simulink model "InjVlv_CalcET1"  (R2016b)
settings: configuration reference "CodeGenConfigSet" (kept outside this file)
values from neighbouring files (symbols this model uses):
  InjVlv_pMin_C = Calibration.Parameter    [init_InjVlv_CalcET.m]    (also in init_InjVlv_CalcET_SIL.m = Simulink.Parameter)
  InjVlv_pMin_CUR = Calibration.Parameter    [init_InjVlv_CalcET.m]    (also in init_InjVlv_CalcET_SIL.m = Simulink.Parameter)
  InjVlv_pMin_CURX = Calibration.Parameter    [init_InjVlv_CalcET.m]    (also in init_InjVlv_CalcET_SIL.m = Simulink.Parameter)
  InjVlv_qMI1Min_CUR = Calibration.Parameter    [init_InjVlv_CalcET.m]    (also in init_InjVlv_CalcET_SIL.m = Simulink.Parameter)
  InjVlv_qMI1Min_CURX = Calibration.Parameter    [init_InjVlv_CalcET.m]    (also in init_InjVlv_CalcET_SIL.m = Simulink.Parameter)
  InjVlv_qPiI1Min_CUR = Calibration.Parameter    [init_InjVlv_CalcET.m]    (also in init_InjVlv_CalcET_SIL.m = Simulink.Parameter)
  InjVlv_qPiI1Min_CURX = Calibration.Parameter    [init_InjVlv_CalcET.m]    (also in init_InjVlv_CalcET_SIL.m = Simulink.Parameter)
  InjVlv_qPiI2Min_CUR = Calibration.Parameter    [init_InjVlv_CalcET.m]    (also in init_InjVlv_CalcET_SIL.m = Simulink.Parameter)
  InjVlv_qPiI2Min_CURX = Calibration.Parameter    [init_InjVlv_CalcET.m]    (also in init_InjVlv_CalcET_SIL.m = Simulink.Parameter)
  InjVlv_qPoI2Min_CUR = Calibration.Parameter    [init_InjVlv_CalcET.m]    (also in init_InjVlv_CalcET_SIL.m = Simulink.Parameter)
  InjVlv_qPoI2Min_CURX = Calibration.Parameter    [init_InjVlv_CalcET.m]    (also in init_InjVlv_CalcET_SIL.m = Simulink.Parameter)
  InjVlv_tiCloseDelay_MAP = Calibration.Parameter    [init_InjVlv_CalcET.m]    (also in init_InjVlv_CalcET_SIL.m = Simulink.Parameter)
  InjVlv_tiCloseDelay_MAPX = Calibration.Parameter    [init_InjVlv_CalcET.m]    (also in init_InjVlv_CalcET_SIL.m = Simulink.Parameter)
  InjVlv_tiCloseDelay_MAPY = Calibration.Parameter    [init_InjVlv_CalcET.m]    (also in init_InjVlv_CalcET_SIL.m = Simulink.Parameter)
  InjVlv_tiDiffMin_MAP = Calibration.Parameter    [init_InjVlv_CalcET.m]    (also in init_InjVlv_CalcET_SIL.m = Simulink.Parameter)
  InjVlv_tiDiffMin_MAPX = Calibration.Parameter    [init_InjVlv_CalcET.m]    (also in init_InjVlv_CalcET_SIL.m = Simulink.Parameter)
  InjVlv_tiDiffMin_MAPY = Calibration.Parameter    [init_InjVlv_CalcET.m]    (also in init_InjVlv_CalcET_SIL.m = Simulink.Parameter)
  InjVlv_tiET_MAP = Calibration.Parameter    [init_InjVlv_CalcET.m]    (also in init_InjVlv_CalcET_SIL.m = Simulink.Parameter)
  InjVlv_tiET_MAPX = Calibration.Parameter    [init_InjVlv_CalcET.m]    (also in init_InjVlv_CalcET_SIL.m = Simulink.Parameter)
  InjVlv_tiET_MAPY = Calibration.Parameter    [init_InjVlv_CalcET.m]    (also in init_InjVlv_CalcET_SIL.m = Simulink.Parameter)
  InjVlv_tiOpenDelay_MAP = Calibration.Parameter    [init_InjVlv_CalcET.m]    (also in init_InjVlv_CalcET_SIL.m = Simulink.Parameter)
  InjVlv_tiOpenDelay_MAPX = Calibration.Parameter    [init_InjVlv_CalcET.m]    (also in init_InjVlv_CalcET_SIL.m = Simulink.Parameter)
  InjVlv_tiOpenDelay_MAPY = Calibration.Parameter    [init_InjVlv_CalcET.m]    (also in init_InjVlv_CalcET_SIL.m = Simulink.Parameter)
  InjVlv_tiPseElec = Calibration.Parameter    [init_InjVlv_CalcET.m]    (also in init_InjVlv_CalcET_SIL.m = Simulink.Parameter)
  SigTst_swtMI1ET_C = Calibration.Parameter    [init_InjVlv_CalcET.m]    (also in init_InjVlv_CalcET_SIL.m = Simulink.Parameter)
  SigTst_swtPiI1ET_C = Calibration.Parameter    [init_InjVlv_CalcET.m]    (also in init_InjVlv_CalcET_SIL.m = Simulink.Parameter)
  SigTst_swtPiI2ET_C = Calibration.Parameter    [init_InjVlv_CalcET.m]    (also in init_InjVlv_CalcET_SIL.m = Simulink.Parameter)
  SigTst_swtPOI2ET_C = Calibration.Parameter    [init_InjVlv_CalcET.m]    (also in init_InjVlv_CalcET_SIL.m = Simulink.Parameter)
  SigTst_tiMI1ET_C = Calibration.Parameter    [init_InjVlv_CalcET.m]    (also in init_InjVlv_CalcET_SIL.m = Simulink.Parameter)
  SigTst_tiPiI1ET_C = Calibration.Parameter    [init_InjVlv_CalcET.m]    (also in init_InjVlv_CalcET_SIL.m = Simulink.Parameter)
  SigTst_tiPiI2ET_C = Calibration.Parameter    [init_InjVlv_CalcET.m]    (also in init_InjVlv_CalcET_SIL.m = Simulink.Parameter)
  SigTst_tiPOI2ET_C = Calibration.Parameter    [init_InjVlv_CalcET.m]    (also in init_InjVlv_CalcET_SIL.m = Simulink.Parameter)
undefined symbols (not defined in the file or in its folder): CEngDst_switch_conv, Switch_conv
libraries: simulink x1
settings Model: Creator=Administrator  LastModifiedBy=mayongchao
settings ConfigSetRef: SourceLocation=Base Workspace

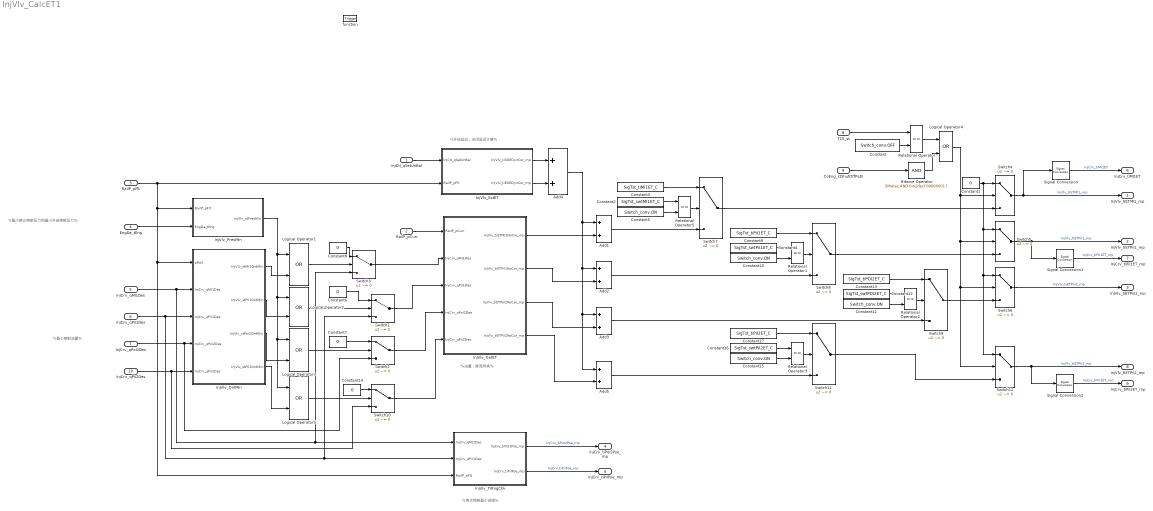
== system InjVlv_CalcET1 ==
  note: %两次喷射最小间隔%
  note: %最小喷射油量%
  note: %最小禁止喷射压力和最小开启喷射压力%
  note: %油量，脉宽转换%
  note: %开启延迟，关闭延迟计算%
  InjCtl_qSetUnBal : Inport  Tag=mg/hub  Description=Current injection quantity  OutMin=-319  OutMax=319  OutDataTypeStr=FuelMass_mg_hub
  RailP_pCurr : Inport  Tag=bar  Description=Current fuel pressure  Port=2  OutMin=0  OutMax=2500  OutDataTypeStr=RailPressure_bar
  RailP_pFlt : Inport  Tag=bar  Description=Maximum rail pressure of the last 10 sampling cycle  Port=3  OutMin=0  OutMax=2500  OutDataTypeStr=RailPressure_bar
  EngDa_tEng : Inport  Tag=deg  Description=Engine temperature  Port=4  OutMin=-1000  OutMax=1000  OutDataTypeStr=Temp_deg
  InjCrv_qMI1Des : Inport  Tag=mg/hub  Description=desired MI1 injection quantity  Port=5  OutMin=-319  OutMax=319  OutDataTypeStr=FuelMass_mg_hub
  InjCrv_qPiI1Des : Inport  Tag=mg/hub  Description=Desired PiI injection quantity  Port=6  OutMin=-319  OutMax=319  OutDataTypeStr=FuelMass_mg_hub
  InjCrv_qPoI2Des : Inport  Tag=mg/hub  Description=Desired PoI2 injection quantity  Port=7  OutMin=-319  OutMax=319  OutDataTypeStr=FuelMass_mg_hub
  T15_st : Inport  Description=Terminal 15 status after debouncing  Port=8  OutDataTypeStr=Enum: Switch_conv
  CoEng_stShutOffPath : Inport  Description=Active shut-off paths resulting from active reversible,irreversible and afterrun shut-off paths  Port=9  OutMin=0  OutMax=65535  OutDataTypeStr=State_uint16
  InjCrv_qPiI2Des : Inport  Tag=mg/hub  Description=Desired PiI injection quantity  Port=10  OutMin=-319  OutMax=319  OutDataTypeStr=FuelMass_mg_hub
  function : TriggerPort  TriggerType=function-call  VariantControl=Variant
  Add{1..5} (5 alike) : Sum  OutDataTypeStr=Inherit: Inherit via back propagation  SaturateOnIntegerOverflow=on  InputSameDT=on
  Bitwise Operator : simulink/Logic and Bit Operations/Bitwise Operator  logicop=AND  UseBitMask=on  BitMask=bin2dec('00000001')  BitMaskRealWorld=Stored Integer
  Constant : Constant  Value=Switch_conv.OFF
  Constant{1,6..8,14} (5 alike) : Constant  Value=0  OutDataTypeStr=Inherit: Inherit via back propagation
  Constant{5,10..11,15} (4 alike) : Constant  Value=Switch_conv.ON  OutDataTypeStr=Inherit: Inherit via back propagation
  Constant12 : Constant  Value=SigTst_swtPOI2ET_C  SampleTime=-1
  Constant13 : Constant  Value=SigTst_tiPOI2ET_C  SampleTime=-1
  Constant16 : Constant  Value=SigTst_swtPiI2ET_C  SampleTime=-1
  Constant17 : Constant  Value=SigTst_tiPiI2ET_C  SampleTime=-1
  Constant2 : Constant  Value=SigTst_swtMI1ET_C  SampleTime=-1
  Constant3 : Constant  Value=SigTst_tiMI1ET_C  SampleTime=-1
  Constant4 : Constant  Value=SigTst_swtPiI1ET_C  SampleTime=-1
  Constant9 : Constant  Value=SigTst_tiPiI1ET_C  SampleTime=-1
  InjVlv_EstET : Subsystem
  InjVlv_GetET : Subsystem
  InjVlv_PresMin : Subsystem
  InjVlv_QntMin : Subsystem
  InjVlv_TiRngChk : Subsystem
  Logical Operator{1..5} (5 alike) : Logic  Operator=OR  AllPortsSameDT=off  OutDataTypeStr=boolean
  Relational Operator : RelationalOperator  Operator===  OutDataTypeStr=boolean  RndMeth=Simplest
  Relational Operator{1..3,5} (4 alike) : RelationalOperator  Operator===  OutDataTypeStr=boolean  RndMeth=Simplest  InputSameDT=on
  Signal Conversion : SignalConversion  OverrideOpt=off
  Signal Conversion1 : SignalConversion  OverrideOpt=off
  Signal Conversion2 : SignalConversion  OverrideOpt=off
  Switch{1..6,10,12} (8 alike) : Switch  Criteria=u2 ~= 0  InputSameDT=on
  Switch{7..9,11} (4 alike) : Switch  Criteria=u2 ~= 0  Threshold=CEngDst_switch_conv.OFF  InputSameDT=on
  InjVlv_tiETMI1_mp : Outport  Tag=us  Description=Start of energizing for MI1  OutMin=-13107  OutMax=13106  OutDataTypeStr=InjTime_us
  InjVlv_tiETPiI1_mp : Outport  Tag=us  Description=Start of energizing for PiI1  Port=2  OutMin=-13107  OutMax=13106  OutDataTypeStr=InjTime_us
  InjVlv_tiETPoI2_mp : Outport  Tag=us  Description=Start of energizing for PoI2  Port=3  OutMin=-13107  OutMax=13106  OutDataTypeStr=InjTime_us
  InjCrv_tiPoI2Pse_mp : Outport  Tag=us  Description=Minium injection interval between MI1 and PoI2  Port=4  OutMin=-13107  OutMax=13106  OutDataTypeStr=InjTime_us
  InjCrv_tiPiIPse_mp : Outport  Tag=us  Description=Minium injection interval between MI1 and PiI1  Port=5  OutMin=-13107  OutMax=13106  OutDataTypeStr=InjTime_us
  InjCrv_tiMI1ET : Outport  Tag=us  Description=Estimated MI1 energizing time  Port=6  OutMin=-13107  OutMax=13106  OutDataTypeStr=InjTime_us
  InjCrv_tiPiI1ET_mp : Outport  Tag=us  Description=Estimated energizing time for PiI1  Port=7  OutMin=-13107  OutMax=13106  OutDataTypeStr=InjTime_us
  InjVlv_tiETPiI2_mp : Outport  Tag=us  Description=Start of energizing for PiI2  Port=8  OutMin=-13107  OutMax=13106  OutDataTypeStr=InjTime_us
  InjCrv_tiPiI2ET_mp : Outport  Tag=us  Description=Estimated energizing time for PiI2  Port=9  OutMin=-13107  OutMax=13106  OutDataTypeStr=InjTime_us
  wires:
  RailP_pFlt/1 -> InjVlv_PresMin/1(RailP_pFlt), InjVlv_TiRngChk/3(RailP_pFlt), InjVlv_QntMin/1(pRail), InjVlv_EstET/2(RailP_pFlt)
  InjCrv_qMI1Des/1 -> Switch3/3, InjVlv_TiRngChk/1(InjCrv_qMI1Des), InjVlv_QntMin/2(InjCrv_qMI1Des)
  Logical Operator1/1 -> Switch3/2
  Constant8/1 -> Switch3/1
  InjVlv_PresMin/1(InjVlv_stPresMin) -> Logical Operator5/1, Logical Operator3/1, Logical Operator2/1, Logical Operator1/1
  InjVlv_QntMin/1(InjVlv_stMI1QntMin) -> Logical Operator1/2
  InjCrv_qPoI2Des/1 -> InjVlv_QntMin/4(InjCrv_qPoI2Des), Switch2/3
  EngDa_tEng/1 -> InjVlv_PresMin/2(EngDa_tEng)
  Switch3/1 -> InjVlv_GetET/2(InjCrv_qMI1Des)
  Constant6/1 -> Switch1/1
  Logical Operator2/1 -> Switch1/2
  InjVlv_QntMin/2(InjVlv_stPiI1QntMin) -> Logical Operator2/2
  Constant7/1 -> Switch2/1
  Logical Operator3/1 -> Switch2/2
  InjVlv_QntMin/3(InjVlv_stPoI2QntMin) -> Logical Operator3/2
  Switch1/1 -> InjVlv_GetET/3(InjCrv_qPiI1Des)
  Switch2/1 -> InjVlv_GetET/4(InjCrv_qPoI2Des)
  InjCtl_qSetUnBal/1 -> InjVlv_EstET/1(InjCtl_qSetUnBal)
  InjVlv_EstET/1(InjVlv_tiSOEDynCor_mp) -> Add4/1
  InjVlv_EstET/2(InjVlv_tiEOEDynCor_mp) -> Add4/2
  InjVlv_GetET/1(InjVlv_tiETMI1NoCor_mp) -> Add1/2
  Add4/1 -> Add5/1, Add3/1, Add2/1, Add1/1
  InjVlv_GetET/2(InjVlv_tiETPiI1NoCor_mp) -> Add2/2
  InjVlv_GetET/3(InjVlv_tiETPoI2NoCor_mp) -> Add3/2
  InjCrv_qPiI1Des/1 -> Switch1/3, InjVlv_TiRngChk/2(InjCrv_qPiI1Des), InjVlv_QntMin/3(InjCrv_qPiI1Des)
  InjVlv_TiRngChk/1(InjCrv_tiPoI2Pse_mp) -> InjCrv_tiPoI2Pse_mp/1  "InjCrv_tiPoI2Pse_mp"
  InjVlv_TiRngChk/2(InjCrv_tiPiIPse_mp) -> InjCrv_tiPiIPse_mp/1  "InjCrv_tiPiIPse_mp"
  RailP_pCurr/1 -> InjVlv_GetET/1(RailP_pCurr)
  Signal Conversion/1 -> InjCrv_tiMI1ET/1  "InjCrv_tiMI1ET"
  Signal Conversion1/1 -> InjCrv_tiPiI1ET_mp/1  "InjCrv_tiPiI1ET_mp"
  T15_st/1 -> Relational Operator/1
  Constant/1 -> Relational Operator/2
  Constant1/1 -> Switch12/1, Switch6/1, Switch5/1, Switch4/1
  Switch4/1 -> Signal Conversion/1, InjVlv_tiETMI1_mp/1  "InjVlv_tiETMI1_mp"
  Relational Operator/1 -> Logical Operator4/1
  Logical Operator4/1 -> Switch12/2, Switch6/2, Switch5/2, Switch4/2
  CoEng_stShutOffPath/1 -> Bitwise Operator/1
  Bitwise Operator/1 -> Logical Operator4/2
  Switch5/1 -> Signal Conversion1/1, InjVlv_tiETPiI1_mp/1  "InjVlv_tiETPiI1_mp"
  Switch6/1 -> InjVlv_tiETPoI2_mp/1  "InjVlv_tiETPoI2_mp"
  Constant3/1 -> Switch7/1
  Relational Operator5/1 -> Switch7/2
  Constant2/1 -> Relational Operator5/1
  Constant5/1 -> Relational Operator5/2
  Add1/1 -> Switch7/3
  Switch7/1 -> Switch4/3
  Constant9/1 -> Switch8/1
  Relational Operator1/1 -> Switch8/2
  Constant4/1 -> Relational Operator1/1
  Constant10/1 -> Relational Operator1/2
  Add2/1 -> Switch8/3
  Switch8/1 -> Switch5/3
  Constant13/1 -> Switch9/1
  Relational Operator2/1 -> Switch9/2
  Constant12/1 -> Relational Operator2/1
  Constant11/1 -> Relational Operator2/2
  Add3/1 -> Switch9/3
  Switch9/1 -> Switch6/3
  InjCrv_qPiI2Des/1 -> Switch10/3, InjVlv_QntMin/5(InjCrv_qPiI2Des)
  InjVlv_QntMin/4(InjVlv_stPiI2QntMin) -> Logical Operator5/2
  Logical Operator5/1 -> Switch10/2
  Constant14/1 -> Switch10/1
  Switch10/1 -> InjVlv_GetET/5(InjCrv_qPiI2Des)
  InjVlv_GetET/4(InjVlv_tiETPiI2NoCor_mp) -> Add5/2
  Add5/1 -> Switch11/3
  Constant17/1 -> Switch11/1
  Relational Operator3/1 -> Switch11/2
  Constant16/1 -> Relational Operator3/1
  Constant15/1 -> Relational Operator3/2
  Switch12/1 -> Signal Conversion2/1, InjVlv_tiETPiI2_mp/1  "InjVlv_tiETPiI2_mp"
  Switch11/1 -> Switch12/3
  Signal Conversion2/1 -> InjCrv_tiPiI2ET_mp/1  "InjCrv_tiPiI2ET_mp"

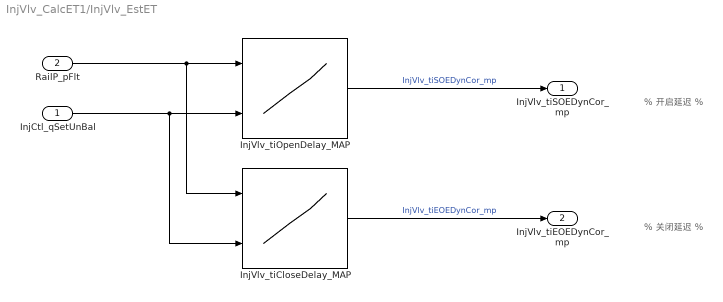
== system InjVlv_CalcET1/InjVlv_EstET ==
  note: % 开启延迟 %
  note: % 关闭延迟 %
  InjCtl_qSetUnBal : Inport
  RailP_pFlt : Inport  Port=2
  InjVlv_tiCloseDelay_MAP : Lookup_n-D  BreakpointsForDimension1=InjVlv_tiCloseDelay_MAPY  BreakpointsForDimension2=InjVlv_tiCloseDelay_MAPX  IndexSearchMethod=Linear search  BeginIndexSearchUsingPreviousIndexResult=on  Table=InjVlv_tiCloseDelay_MAP  ExtrapMethod=Clip  UseLastTableValue=on  InternalRulePriority=Speed  OutDataTypeStr=Inherit: Inherit via back propagation  SaturateOnIntegerOverflow=on
  InjVlv_tiOpenDelay_MAP : Lookup_n-D  BreakpointsForDimension1=InjVlv_tiOpenDelay_MAPY  BreakpointsForDimension2=InjVlv_tiOpenDelay_MAPX  IndexSearchMethod=Linear search  BeginIndexSearchUsingPreviousIndexResult=on  Table=InjVlv_tiOpenDelay_MAP  ExtrapMethod=Clip  UseLastTableValue=on  InternalRulePriority=Speed  OutDataTypeStr=Inherit: Inherit via back propagation  SaturateOnIntegerOverflow=on
  InjVlv_tiSOEDynCor_mp : Outport
  InjVlv_tiEOEDynCor_mp : Outport  Port=2
  wires:
  RailP_pFlt/1 -> InjVlv_tiCloseDelay_MAP/1, InjVlv_tiOpenDelay_MAP/1
  InjCtl_qSetUnBal/1 -> InjVlv_tiCloseDelay_MAP/2, InjVlv_tiOpenDelay_MAP/2
  InjVlv_tiCloseDelay_MAP/1 -> InjVlv_tiEOEDynCor_mp/1  "InjVlv_tiEOEDynCor_mp"
  InjVlv_tiOpenDelay_MAP/1 -> InjVlv_tiSOEDynCor_mp/1  "InjVlv_tiSOEDynCor_mp"

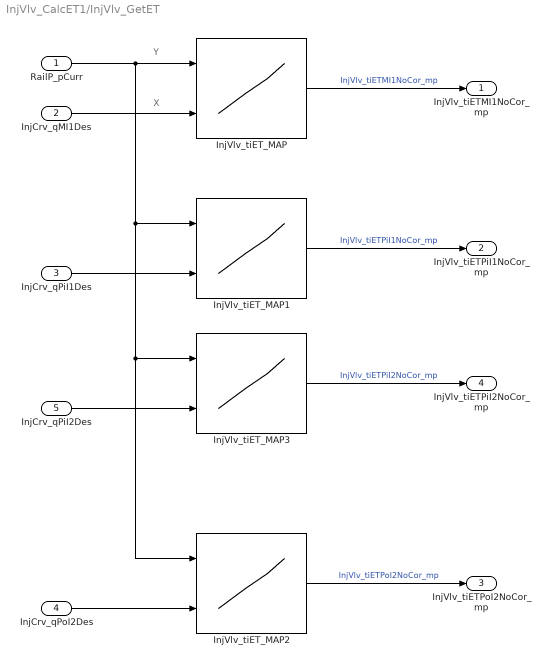
== system InjVlv_CalcET1/InjVlv_GetET ==
  note: Y
  note: X
  RailP_pCurr : Inport
  InjCrv_qMI1Des : Inport  Port=2
  InjCrv_qPiI1Des : Inport  Port=3
  InjCrv_qPoI2Des : Inport  Port=4
  InjCrv_qPiI2Des : Inport  Port=5
  InjVlv_tiET_MAP{,1..3} (4 alike) : Lookup_n-D  BreakpointsForDimension1=InjVlv_tiET_MAPY  BreakpointsForDimension2=InjVlv_tiET_MAPX  IndexSearchMethod=Linear search  BeginIndexSearchUsingPreviousIndexResult=on  Table=InjVlv_tiET_MAP  ExtrapMethod=Clip  UseLastTableValue=on  InternalRulePriority=Speed  OutDataTypeStr=Inherit: Inherit via back propagation  SaturateOnIntegerOverflow=on
  InjVlv_tiETMI1NoCor_mp : Outport
  InjVlv_tiETPiI1NoCor_mp : Outport  Port=2
  InjVlv_tiETPoI2NoCor_mp : Outport  Port=3
  InjVlv_tiETPiI2NoCor_mp : Outport  Port=4
  wires:
  InjCrv_qMI1Des/1 -> InjVlv_tiET_MAP/2
  InjCrv_qPiI1Des/1 -> InjVlv_tiET_MAP1/2
  InjCrv_qPoI2Des/1 -> InjVlv_tiET_MAP2/2
  InjVlv_tiET_MAP/1 -> InjVlv_tiETMI1NoCor_mp/1  "InjVlv_tiETMI1NoCor_mp"
  InjVlv_tiET_MAP1/1 -> InjVlv_tiETPiI1NoCor_mp/1  "InjVlv_tiETPiI1NoCor_mp"
  InjVlv_tiET_MAP2/1 -> InjVlv_tiETPoI2NoCor_mp/1  "InjVlv_tiETPoI2NoCor_mp"
  RailP_pCurr/1 -> InjVlv_tiET_MAP1/1, InjVlv_tiET_MAP3/1, InjVlv_tiET_MAP2/1, InjVlv_tiET_MAP/1
  InjCrv_qPiI2Des/1 -> InjVlv_tiET_MAP3/2
  InjVlv_tiET_MAP3/1 -> InjVlv_tiETPiI2NoCor_mp/1  "InjVlv_tiETPiI2NoCor_mp"

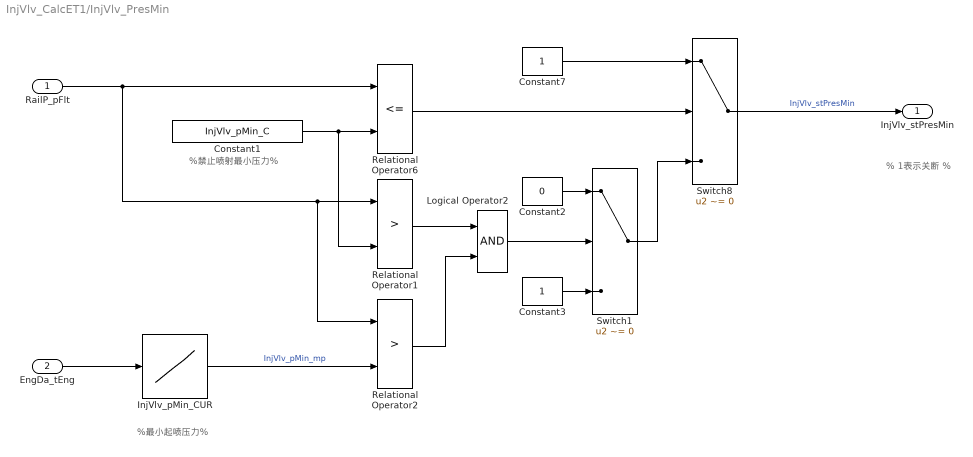
== system InjVlv_CalcET1/InjVlv_PresMin ==
  note: % 1表示关断 %
  note: %禁止喷射最小压力%
  note: %最小起喷压力%
  RailP_pFlt : Inport
  EngDa_tEng : Inport  Port=2
  Constant1 : Constant  Value=InjVlv_pMin_C
  Constant2 : Constant  Value=0  OutDataTypeStr=boolean
  Constant3 : Constant  OutDataTypeStr=boolean
  Constant7 : Constant  OutDataTypeStr=boolean
  InjVlv_pMin_CUR : Lookup_n-D  NumberOfTableDimensions=1  BreakpointsForDimension1=InjVlv_pMin_CURX  BreakpointsForDimension3=[5, 7]  IndexSearchMethod=Linear search  BeginIndexSearchUsingPreviousIndexResult=on  Table=InjVlv_pMin_CUR  ExtrapMethod=Clip  UseLastTableValue=on  InternalRulePriority=Speed  OutDataTypeStr=Inherit: Inherit via back propagation  SaturateOnIntegerOverflow=on
  Logical Operator2 : Logic  OutDataTypeStr=boolean
  Relational Operator1 : RelationalOperator  Operator=>  OutDataTypeStr=boolean  RndMeth=Round  InputSameDT=on
  Relational Operator2 : RelationalOperator  Operator=>  OutDataTypeStr=boolean  RndMeth=Round  InputSameDT=on
  Relational Operator6 : RelationalOperator  Operator=<=  OutDataTypeStr=boolean  RndMeth=Round  InputSameDT=on
  Switch1 : Switch  Criteria=u2 ~= 0  OutDataTypeStr=Inherit: Inherit via back propagation  RndMeth=Round  InputSameDT=on
  Switch8 : Switch  Criteria=u2 ~= 0  OutDataTypeStr=Inherit: Inherit via back propagation  RndMeth=Round  InputSameDT=on
  InjVlv_stPresMin : Outport
  wires:
  EngDa_tEng/1 -> InjVlv_pMin_CUR/1
  InjVlv_pMin_CUR/1 -> Relational Operator2/2  "InjVlv_pMin_mp"
  RailP_pFlt/1 -> Relational Operator1/1, Relational Operator2/1, Relational Operator6/1
  Constant7/1 -> Switch8/1
  Switch8/1 -> InjVlv_stPresMin/1  "InjVlv_stPresMin"
  Constant1/1 -> Relational Operator1/2, Relational Operator6/2
  Relational Operator6/1 -> Switch8/2
  Switch1/1 -> Switch8/3
  Logical Operator2/1 -> Switch1/2
  Relational Operator1/1 -> Logical Operator2/1
  Relational Operator2/1 -> Logical Operator2/2
  Constant2/1 -> Switch1/1
  Constant3/1 -> Switch1/3

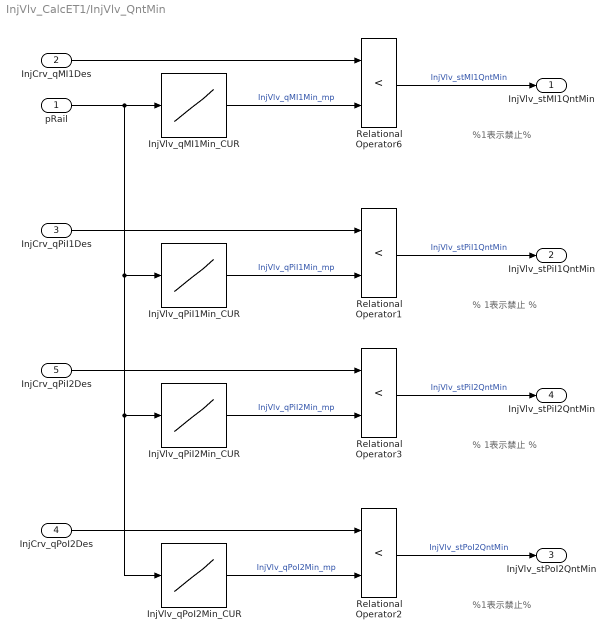
== system InjVlv_CalcET1/InjVlv_QntMin ==
  note: %1表示禁止%
  note: % 1表示禁止 %
  note: %1表示禁止%
  note: % 1表示禁止 %
  pRail : Inport
  InjCrv_qMI1Des : Inport  Port=2
  InjCrv_qPiI1Des : Inport  Port=3
  InjCrv_qPoI2Des : Inport  Port=4
  InjCrv_qPiI2Des : Inport  Port=5
  InjVlv_qMI1Min_CUR : Lookup_n-D  NumberOfTableDimensions=1  BreakpointsForDimension1=InjVlv_qMI1Min_CURX  BreakpointsForDimension3=[5, 7]  IndexSearchMethod=Linear search  BeginIndexSearchUsingPreviousIndexResult=on  Table=InjVlv_qMI1Min_CUR  ExtrapMethod=Clip  UseLastTableValue=on  InternalRulePriority=Speed  OutDataTypeStr=Inherit: Inherit via back propagation  SaturateOnIntegerOverflow=on
  InjVlv_qPiI1Min_CUR : Lookup_n-D  NumberOfTableDimensions=1  BreakpointsForDimension1=InjVlv_qPiI1Min_CURX  BreakpointsForDimension3=[5, 7]  IndexSearchMethod=Linear search  BeginIndexSearchUsingPreviousIndexResult=on  Table=InjVlv_qPiI1Min_CUR  ExtrapMethod=Clip  UseLastTableValue=on  InternalRulePriority=Speed  OutDataTypeStr=Inherit: Inherit via back propagation  SaturateOnIntegerOverflow=on
  InjVlv_qPiI2Min_CUR : Lookup_n-D  NumberOfTableDimensions=1  BreakpointsForDimension1=InjVlv_qPiI2Min_CURX  BreakpointsForDimension3=[5, 7]  IndexSearchMethod=Linear search  BeginIndexSearchUsingPreviousIndexResult=on  Table=InjVlv_qPiI2Min_CUR  ExtrapMethod=Clip  UseLastTableValue=on  InternalRulePriority=Speed  OutDataTypeStr=Inherit: Inherit via back propagation  SaturateOnIntegerOverflow=on
  InjVlv_qPoI2Min_CUR : Lookup_n-D  NumberOfTableDimensions=1  BreakpointsForDimension1=InjVlv_qPoI2Min_CURX  BreakpointsForDimension3=[5, 7]  IndexSearchMethod=Linear search  BeginIndexSearchUsingPreviousIndexResult=on  Table=InjVlv_qPoI2Min_CUR  ExtrapMethod=Clip  UseLastTableValue=on  InternalRulePriority=Speed  OutDataTypeStr=Inherit: Inherit via back propagation  SaturateOnIntegerOverflow=on
  Relational Operator{1..3,6} (4 alike) : RelationalOperator  Operator=<  OutDataTypeStr=boolean  RndMeth=Round  InputSameDT=on
  InjVlv_stMI1QntMin : Outport
  InjVlv_stPiI1QntMin : Outport  Port=2
  InjVlv_stPoI2QntMin : Outport  Port=3
  InjVlv_stPiI2QntMin : Outport  Port=4
  wires:
  InjVlv_qMI1Min_CUR/1 -> Relational Operator6/2  "InjVlv_qMI1Min_mp"
  InjCrv_qMI1Des/1 -> Relational Operator6/1
  Relational Operator6/1 -> InjVlv_stMI1QntMin/1  "InjVlv_stMI1QntMin"
  Relational Operator1/1 -> InjVlv_stPiI1QntMin/1  "InjVlv_stPiI1QntMin"
  InjCrv_qPiI1Des/1 -> Relational Operator1/1
  InjVlv_qPiI1Min_CUR/1 -> Relational Operator1/2  "InjVlv_qPiI1Min_mp"
  InjVlv_qPoI2Min_CUR/1 -> Relational Operator2/2  "InjVlv_qPoI2Min_mp"
  InjCrv_qPoI2Des/1 -> Relational Operator2/1
  Relational Operator2/1 -> InjVlv_stPoI2QntMin/1  "InjVlv_stPoI2QntMin"
  Relational Operator3/1 -> InjVlv_stPiI2QntMin/1  "InjVlv_stPiI2QntMin"
  InjCrv_qPiI2Des/1 -> Relational Operator3/1
  InjVlv_qPiI2Min_CUR/1 -> Relational Operator3/2  "InjVlv_qPiI2Min_mp"
  pRail/1 -> InjVlv_qPiI2Min_CUR/1, InjVlv_qPoI2Min_CUR/1, InjVlv_qPiI1Min_CUR/1, InjVlv_qMI1Min_CUR/1

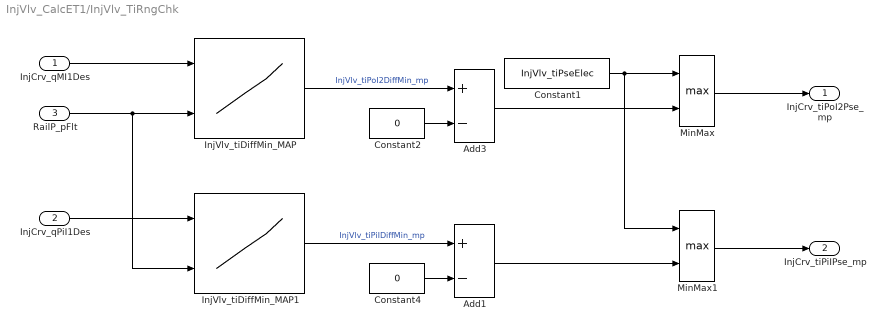
== system InjVlv_CalcET1/InjVlv_TiRngChk ==
  InjCrv_qMI1Des : Inport
  InjCrv_qPiI1Des : Inport  Port=2
  RailP_pFlt : Inport  Port=3
  Add1 : Sum  Inputs=+-  SaturateOnIntegerOverflow=on  InputSameDT=on
  Add3 : Sum  Inputs=+-  SaturateOnIntegerOverflow=on  InputSameDT=on
  Constant1 : Constant  Value=InjVlv_tiPseElec
  Constant2 : Constant  Value=0  OutDataTypeStr=Inherit: Inherit via back propagation
  Constant4 : Constant  Value=0  OutDataTypeStr=Inherit: Inherit via back propagation
  InjVlv_tiDiffMin_MAP : Lookup_n-D  BreakpointsForDimension1=InjVlv_tiDiffMin_MAPY  BreakpointsForDimension2=InjVlv_tiDiffMin_MAPX  IndexSearchMethod=Linear search  BeginIndexSearchUsingPreviousIndexResult=on  Table=InjVlv_tiDiffMin_MAP  ExtrapMethod=Clip  UseLastTableValue=on  InternalRulePriority=Speed  OutDataTypeStr=Inherit: Inherit via back propagation  SaturateOnIntegerOverflow=on
  InjVlv_tiDiffMin_MAP1 : Lookup_n-D  BreakpointsForDimension1=InjVlv_tiDiffMin_MAPY  BreakpointsForDimension2=InjVlv_tiDiffMin_MAPX  IndexSearchMethod=Linear search  BeginIndexSearchUsingPreviousIndexResult=on  Table=InjVlv_tiDiffMin_MAP  ExtrapMethod=Clip  UseLastTableValue=on  InternalRulePriority=Speed  OutDataTypeStr=Inherit: Inherit via back propagation  SaturateOnIntegerOverflow=on
  MinMax : MinMax  Function=max  Inputs=2  OutDataTypeStr=Inherit: Inherit via back propagation  InputSameDT=on
  MinMax1 : MinMax  Function=max  Inputs=2  OutDataTypeStr=Inherit: Inherit via back propagation  InputSameDT=on
  InjCrv_tiPoI2Pse_mp : Outport
  InjCrv_tiPiIPse_mp : Outport  Port=2
  wires:
  MinMax/1 -> InjCrv_tiPoI2Pse_mp/1
  InjCrv_qMI1Des/1 -> InjVlv_tiDiffMin_MAP/1
  InjVlv_tiDiffMin_MAP/1 -> Add3/1  "InjVlv_tiPoI2DiffMin_mp"
  Constant2/1 -> Add3/2
  Add3/1 -> MinMax/2
  MinMax1/1 -> InjCrv_tiPiIPse_mp/1
  InjCrv_qPiI1Des/1 -> InjVlv_tiDiffMin_MAP1/1
  RailP_pFlt/1 -> InjVlv_tiDiffMin_MAP1/2, InjVlv_tiDiffMin_MAP/2
  InjVlv_tiDiffMin_MAP1/1 -> Add1/1  "InjVlv_tiPiIDiffMin_mp"
  Constant4/1 -> Add1/2
  Add1/1 -> MinMax1/2
  Constant1/1 -> MinMax1/1, MinMax/1
